simulink model "MR_STMD_control"  (R2021b)
settings: Solver=VariableStepAuto  StartTime=0.0  StopTime=10.0  RelTol=1e-3
values from neighbouring files (symbols this model uses):
  Kmax = 50*ct    [Run_MdE_Research_Report.m]    (also in my_script.m)
  Kmin = ct/2    [Run_MdE_Research_Report.m]    (also in my_script.m)
  kt = ((2*pi*ft)^2)*mt    [Run_MdE_Research_Report.m]    (also in Run_MdE_Research_Report_con_MR_damper.m; my_script.m)
  mt = mu*m1    (= 0.02)    [Run_MdE_Research_Report.m]    (also in Run_MdE_Research_Report_con_MR_damper.m = 40; my_script.m)
  tend = 500    [Run_MdE_Research_Report.m]    (also in Run_MdE_Research_Report_con_MR_damper.m; my_script.m)
  ts = 1/fs    (= 0.000666666666667)    [Run_MdE_Research_Report.m]    (also in Run_MdE_Research_Report_con_MR_damper.m; my_script.m)
undefined symbols (not defined in the file or in its folder): D_Gs, N_Gs, sigbuilder_block
libraries: simulink x1
settings Model: Creator=luismiguelmartinezgomez  LastModifiedBy=luismiguelmartinezgomez

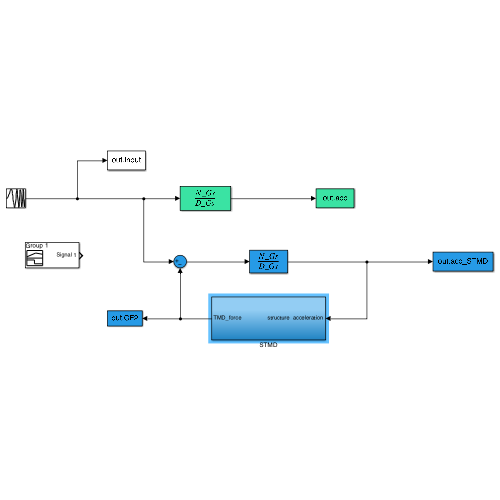
[thumbnail: Simulink's stored preview of the top-level diagram]
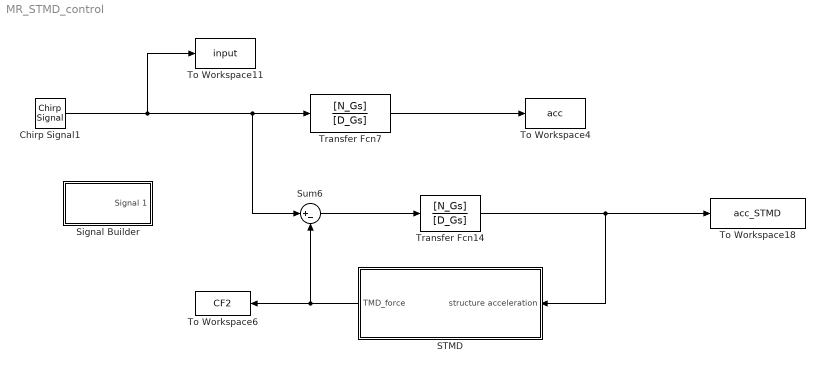
== system MR_STMD_control ==
  Chirp Signal1 : simulink/Sources/Chirp Signal  f1=fmin  T=tend  f2=fmax
  STMD : Subsystem
  Signal Builder : Subsystem  Tag=STV Subsys  LoadFcn=sigbuilder_block('load');  StartFcn=sigbuilder_block('start');  StopFcn=sigbuilder_block('stop');  ClipboardFcn=sigbuilder_block('clipboard');  mask(Sigbuilder block){tuvar=[0:10]}
      mask help: Simulink:masks:SigbuilderBlock_MD
      mask init:
      | if ~strcmp(get_param(bdroot(gcbh),'SimulationStatus'),'stopped') tuvar = sigbuilder_block('maskInit'); end
      settings: CopyFcn=sigbuilder_block('copy');  DeleteFcn=sigbuilder_block('delete');  ModelCloseFcn=sigbuilder_block('modelClose');  PreSaveFcn=sigbuilder_block('preSave');  PauseFcn=sigbuilder_block('pause');  ContinueFcn=sigbuilder_block('continue');  NameChangeFcn=sigbuilder_block('namechange');  OpenFcn=sigbuilder_block('open',[0 0 1440 796 ]);  CloseFcn=sigbuilder_block('close');
      mask Display: plot(0, 0, 100, 100,[2, 2, 32, 32, 2], [68, 8, 8, 68, 68],[32, 2], [38, 38], [32, 19, 2],[53, 60, 44], [32, 17, 17, 2],[16, 16, 31, 31]);txt = getActiveGroup(gcbh);text(2, 100, txt,'verticalAlignment', 'top');
  Sum6 : Sum  Inputs=|+-
  To Workspace11 : ToWorkspace  VariableName=input  SampleTime=ts
  To Workspace18 : ToWorkspace  VariableName=acc_STMD  SampleTime=ts
  To Workspace4 : ToWorkspace  VariableName=acc  SampleTime=ts
  To Workspace6 : ToWorkspace  VariableName=CF2  SampleTime=ts
  Transfer Fcn14 : TransferFcn  Numerator=[N_Gs]  Denominator=[D_Gs]
  Transfer Fcn7 : TransferFcn  Numerator=[N_Gs]  Denominator=[D_Gs]
  wires:
  Transfer Fcn7/1 -> To Workspace4/1
  Transfer Fcn14/1 -> STMD/1(structure acceleration), To Workspace18/1
  Chirp Signal1/1 -> Sum6/1, Transfer Fcn7/1, To Workspace11/1
  Sum6/1 -> Transfer Fcn14/1
  STMD/1(TMD_force) -> To Workspace6/1, Sum6/2

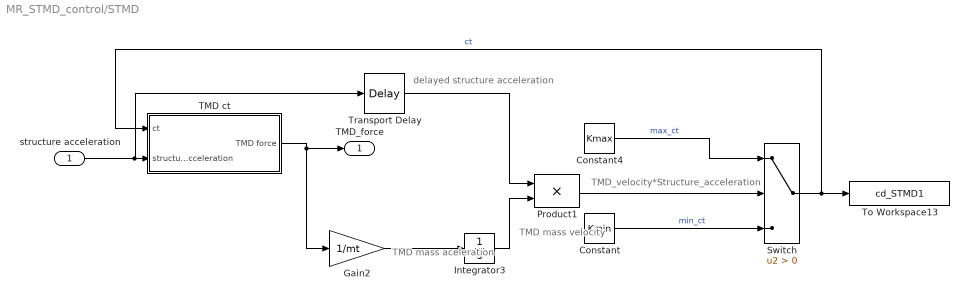
== system MR_STMD_control/STMD ==
  note: delayed structure acceleration
  note: TMD mass
      | aceleration
  note: TMD_velocity*Structure_acceleration
  note: TMD mass
      | velocity
  structure acceleration : Inport
  Constant : Constant  Value=Kmin
  Constant4 : Constant  Value=Kmax
  Gain2 : Gain  Gain=1/mt
  Integrator3 : Integrator
  Product1 : Product  OutDataTypeStr=double  SaturateOnIntegerOverflow=on
  Switch : Switch  Criteria=u2 > Threshold
  TMD ct : Subsystem
  To Workspace13 : ToWorkspace  VariableName=cd_STMD1  SampleTime=ts
  Transport Delay : TransportDelay  DelayTime=ts
  TMD_force : Outport  VectorParamsAs1DForOutWhenUnconnected=off
  wires:
  TMD ct/1(TMD force) -> Gain2/1, TMD_force/1
  Integrator3/1 -> Product1/2
  Switch/1 -> To Workspace13/1, TMD ct/1(ct)  "ct"
  structure acceleration/1 -> Transport Delay/1, TMD ct/2(structure_acceleration)
  Transport Delay/1 -> Product1/1
  Gain2/1 -> Integrator3/1
  Product1/1 -> Switch/2
  Constant4/1 -> Switch/1  "max_ct"
  Constant/1 -> Switch/3  "min_ct"

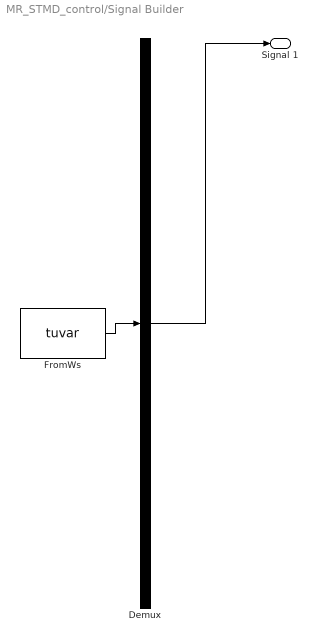
== system MR_STMD_control/Signal Builder ==
  Demux : Demux  Tag=STV Demux  Outputs=1
      settings: DisplayOption=none
  FromWs : FromWorkspace  Tag=STV FromWs  VariableName=tuvar
      SigBuilderData=|
      | common.afterFinalStr = 'Extrapolate'
      | common.sampleTime = 0
      | dataSet.timeRange = [0 10]
      | dataSet.name = 'Group 1'
      | sbobj.Groups.Name = 'Group 1'
      | sbobj.Groups.Signals.Name = 'Signal 1'
      | sbobj.Groups.Signals.XData = [0 4 4 6 6 10]
      | sbobj.Groups.Signals.YData = [0 0 1 1 0 0]
  Signal 1 : Outport  Tag=STV Outport
  wires:
  Demux/1 -> Signal 1/1
  FromWs/1 -> Demux/1

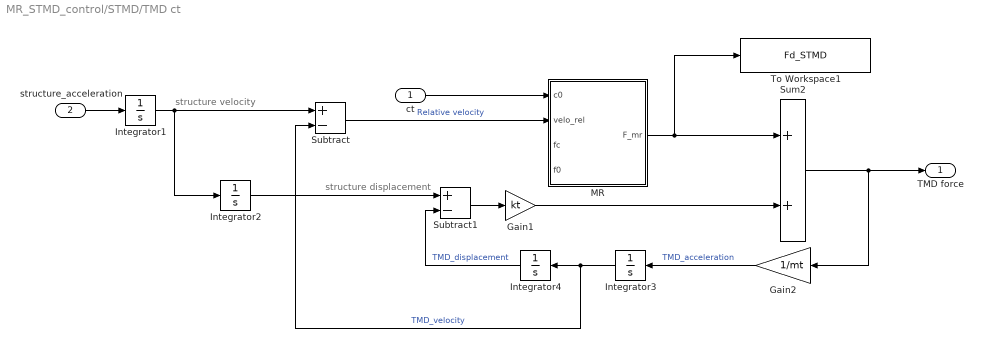
== system MR_STMD_control/STMD/TMD ct ==
  note: structure displacement
  note: structure velocity
  ct : Inport
  structure_acceleration : Inport  Port=2
  Gain1 : Gain  Gain=kt
  Gain2 : Gain  Gain=1/mt
  Integrator{1..4} (4 alike) : Integrator
  MR : Subsystem
  Subtract : Sum  Inputs=+-
  Subtract1 : Sum  Inputs=+-
  Sum2 : Sum
  To Workspace1 : ToWorkspace  VariableName=Fd_STMD  SampleTime=ts
  TMD force : Outport  VectorParamsAs1DForOutWhenUnconnected=off
  wires:
  Integrator1/1 -> Subtract/1, Integrator2/1
  structure_acceleration/1 -> Integrator1/1
  Integrator3/1 -> Subtract/2, Integrator4/1  "TMD_velocity"
  Gain2/1 -> Integrator3/1  "TMD_acceleration"
  Integrator4/1 -> Subtract1/2  "TMD_displacement"
  Integrator2/1 -> Subtract1/1
  Subtract1/1 -> Gain1/1
  Sum2/1 -> TMD force/1, Gain2/1
  ct/1 -> MR/1(c0)
  Subtract/1 -> MR/2(velo_rel)  "Relative velocity"
  MR/1(F_mr) -> To Workspace1/1, Sum2/1
  Gain1/1 -> Sum2/2

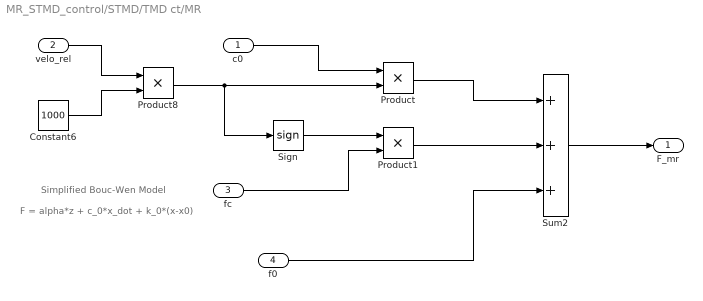
== system MR_STMD_control/STMD/TMD ct/MR ==
  note: Simplified Bouc-Wen Model
  note: F = alpha*z + c_0*x_dot + k_0*(x-x0)
  c0 : Inport
  velo_rel : Inport  Port=2
  "fc " : Inport  Port=3
  f0 : Inport  Port=4
  Constant6 : Constant  Value=1000
  Product : Product
  Product1 : Product
  Product8 : Product
  Sign : Signum
  Sum2 : Sum  Inputs=+++
  F_mr : Outport  VectorParamsAs1DForOutWhenUnconnected=off
  wires:
  velo_rel/1 -> Product8/1
  Constant6/1 -> Product8/2
  c0/1 -> Product/1
  Sum2/1 -> F_mr/1
  Product1/1 -> Sum2/2
  Product/1 -> Sum2/1
  Product8/1 -> Sign/1, Product/2
  "fc "/1 -> Product1/2
  Sign/1 -> Product1/1
  f0/1 -> Sum2/3
